simulink model "req13"  (R2019a)
settings: Solver=FixedStepAuto  StartTime=0.0  StopTime=100  RelTol=1e-3
settings Model: Creator=e40014285  LastModifiedBy=e40014285
settings ConfigComp: CovEnable=on  CovScope=ReferencedModels  RecordCoverage=on  CovHTMLOptions=-sRT=1 -sVT=0 -aTS=1 -bRG=1 -bTC=1 -hTR=0 -nFC=0 -nFD=1 -scm=1 -bcm=1 -xEv=0 -xEM=0  CovHtmlReporting=on  CovCumulativeReport=on  DVModelCoverageObjectives=EnhancedMCDC  DVTestSuiteOptimization=Auto  DVDetectOutOfBounds=on  DVReportPDFFormat=on  DVRebuildModelRepresentation=Always

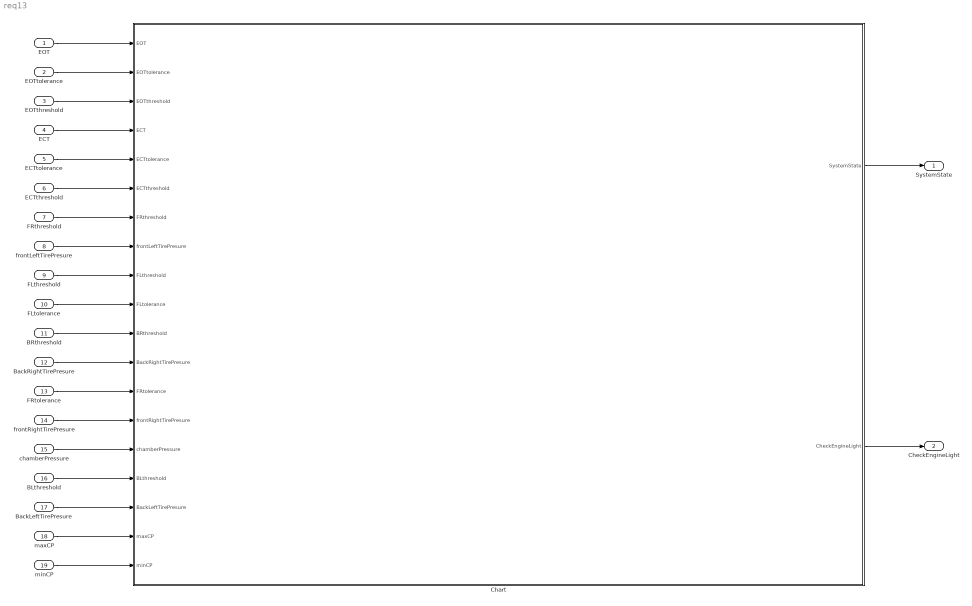
== system req13 ==
  EOT : Inport
  EOTtolerance : Inport  Port=2
  EOTthreshold : Inport  Port=3
  ECT : Inport  Port=4
  ECTtolerance : Inport  Port=5
  ECTthreshold : Inport  Port=6
  FRthreshold : Inport  Port=7
  frontLeftTirePresure : Inport  Port=8
  FLthreshold : Inport  Port=9
  FLtolerance : Inport  Port=10
  BRthreshold : Inport  Port=11
  BackRightTirePresure : Inport  Port=12
  FRtolerance : Inport  Port=13
  frontRightTirePresure : Inport  Port=14
  chamberPressure : Inport  Port=15
  BLthreshold : Inport  Port=16
  BackLeftTirePresure : Inport  Port=17
  maxCP : Inport  Port=18
  minCP : Inport  Port=19
  Chart : Stateflow chart  BlockKeywords=__PRM__SERIALIZED__DATA__:Stateflow Chart,Stateflow Diagram  TreatAsAtomicUnit=on
  SystemState : Outport
  CheckEngineLight : Outport  Port=2
  wires:
  FLthreshold/1 -> Chart/9(FLthreshold)
  chamberPressure/1 -> Chart/15(chamberPressure)
  frontLeftTirePresure/1 -> Chart/8(frontLeftTirePresure)
  FRthreshold/1 -> Chart/7(FRthreshold)
  FLtolerance/1 -> Chart/10(FLtolerance)
  FRtolerance/1 -> Chart/13(FRtolerance)
  BackRightTirePresure/1 -> Chart/12(BackRightTirePresure)
  BRthreshold/1 -> Chart/11(BRthreshold)
  Chart/1(SystemState) -> SystemState/1
  BackLeftTirePresure/1 -> Chart/17(BackLeftTirePresure)
  BLthreshold/1 -> Chart/16(BLthreshold)
  EOTtolerance/1 -> Chart/2(EOTtolerance)
  ECTtolerance/1 -> Chart/5(ECTtolerance)
  frontRightTirePresure/1 -> Chart/14(frontRightTirePresure)
  maxCP/1 -> Chart/18(maxCP)
  EOTthreshold/1 -> Chart/3(EOTthreshold)
  ECT/1 -> Chart/4(ECT)
  Chart/2(CheckEngineLight) -> CheckEngineLight/1
  minCP/1 -> Chart/19(minCP)
  EOT/1 -> Chart/1(EOT)
  ECTthreshold/1 -> Chart/6(ECTthreshold)

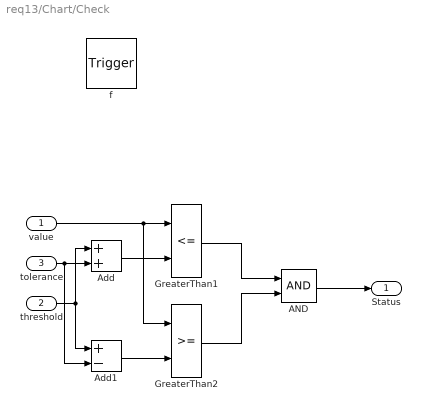
== system req13/Chart/Check ==
  value : Inport  OutDataTypeStr=double  PortDimensions=1
  threshold : Inport  Port=2  OutDataTypeStr=double  PortDimensions=1
  tolerance : Inport  Port=3  OutDataTypeStr=double  PortDimensions=1
  f : TriggerPort  TriggerType=function-call  VariantControl=(inherit)
      settings: CopyFcn=Stateflow.SLINSF.SimulinkMan.removeBlockPreDeleteFcn  PreDeleteFcn=Stateflow.SLINSF.SimulinkMan.unsafePredeleteFcn
  AND : Logic  AllPortsSameDT=off  OutDataTypeStr=boolean
  Add : Sum
  Add1 : Sum  Inputs=+-
  GreaterThan1 : RelationalOperator  Operator=<=  OutDataTypeStr=boolean  RndMeth=Simplest
  GreaterThan2 : RelationalOperator  OutDataTypeStr=boolean  RndMeth=Simplest
  Status : Outport
  wires:
  value/1 -> GreaterThan2/1, GreaterThan1/1
  threshold/1 -> Add/1, Add1/1
  Add/1 -> GreaterThan1/2
  tolerance/1 -> Add1/2, Add/2
  Add1/1 -> GreaterThan2/2
  GreaterThan2/1 -> AND/2
  GreaterThan1/1 -> AND/1
  AND/1 -> Status/1

== stateflow chart req13/Chart ==
  state default
  state Status=Check(value,threshold,tolerance) [function]
  state green
    CheckEngineLight=0;
    SystemState=1;
  state wait
    en:
    time=0;
    exitState=false;
    du:
    time=time+1;
    exitState=(time > 10);
  state orange1
    CheckEngineLight=0;
    SystemState=2;
  state red
    CheckEngineLight=1;
    SystemState=3;
  (default) -> default
  default -> green : [Check(frontRightTirePresure,FRthreshold,FRtolerance)...
      | && Check(frontLeftTirePresure,FLthreshold,FLtolerance)...
      | && Check(BackRightTirePresure,BRthreshold,FRtolerance)...
      | && Check(BackLeftTirePresure,BLthreshold,FLtolerance)...
      | && Check(ECT,ECTthreshold,ECTtolerance)...
      | && Check(EOT,EOTthreshold,EOTtolerance)...
      | && (chamberPressure<maxCP && chamberPressure > minCP)]
  green -> wait : [~Check(frontRightTirePresure,FRthreshold,FRtolerance)...
      | || ~Check(frontLeftTirePresure,FLthreshold,FLtolerance)...
      | || ~Check(BackRightTirePresure,BRthreshold,FRtolerance)...
      | || ~Check(BackLeftTirePresure,BLthreshold,FLtolerance)...
      | || ~Check(ECT,ECTthreshold,ECTtolerance)...
      | || ~Check(EOT,EOTthreshold,EOTtolerance)...
      | || (chamberPressure>=maxCP && chamberPressure <= minCP)]
  wait -> orange1 : [exitState]
  orange1 -> red : [(int8(~Check(frontRightTirePresure,FRthreshold,FRtolerance))...
      | + int8(~Check(frontLeftTirePresure,FLthreshold,FLtolerance))...
      | + int8(~Check(BackRightTirePresure,BRthreshold,FRtolerance))...
      | + int8(~Check(BackLeftTirePresure,BLthreshold,FLtolerance))...
      | + int8(~Check(ECT,ECTthreshold,ECTtolerance))...
      | + int8(~Check(EOT,EOTthreshold,EOTtolerance))...
      | + int8((chamberPressure>=maxCP && chamberPressure <= minCP)))>=2]
  data: value function_input double size=1; threshold function_input double size=1; Status function_output; tolerance function_input double size=1; EOT input; EOTtolerance input; EOTthreshold input; ECT input; ECTtolerance input; ECTthreshold input; FRthreshold input; frontLeftTirePresure input; FLthreshold input; FLtolerance input; BRthreshold input; BackRightTirePresure input; FRtolerance input; frontRightTirePresure input; chamberPressure input; BLthreshold input; BackLeftTirePresure input; maxCP input; minCP input; SystemState output; CheckEngineLight output; exitState local; time local
